simulink model "test_without_actuator"  (R2022b)
settings: Solver=FixedStepAuto  StartTime=0.0  StopTime=10  FixedStep=0.1  RelTol=1e-3
values from neighbouring files (symbols this model uses):
  C_M = 1.1366    [init.m]
  C_T = 3.5611    [init.m]
  D_p = 0.1    [init.m]
  model_param = struct(     'I', I,      'mass', ModelParam_m,      'g', ModelParam_g,      'c_T', ModelParam_c_T,      'c_M', ModelParam_c_M,      'd', ModelParam_d,      'J_RP', ModelParam_J_RP,      'init_pos', [ModelInit_Pos_x, ModelInit_Pos_y, ModelInit_Pos_z],      'init_att', [ModelInit_Att_x, ModelInit_Att_y, ModelInit_Att_z],      'C_T', C_T,      'C_M', C_M,      'air_density', p,      'prop_diameter',  ...(+52 chars)    [init.m]
  ModelInit_Att_qw = 0    [init.m]
  ModelInit_Att_qx = 1    [init.m]
  ModelInit_Att_qy = 0    [init.m]
  ModelInit_Att_qz = 0    [init.m]
  ModelInit_Pos_x = 0    [init.m]
  ModelInit_Pos_y = 0    [init.m]
  ModelInit_Pos_z = 0    [init.m]
  ModelParam_c_M = 1.779e-07*2    (= 3.558e-07)    [init.m]
  ModelParam_c_T = 1.105e-05    [init.m]
  ModelParam_d = 0.225    [init.m]
  ModelParam_g = 9.8    [init.m]
  ModelParam_I_xx = 0.0211    [init.m]
  ModelParam_I_yy = 0.0219    [init.m]
  ModelParam_I_zz = 0.0366    [init.m]
  ModelParam_J_RP = 0.0001287    [init.m]
  ModelParam_m = 1.4    [init.m]
  p = pos(idx,:)    [draw_morecool.m]    (also in init.m = 1.225)
(part 2 of 2)

== system test_without_actuator/混合无人机模型1/Quadcopter Dynamics Model/Rigid-Body Kinematic Model/Attitude Kinematic Model1 ==
  p : Inport
  q : Inport  Port=2
  r : Inport  Port=3
  Constant1 : Constant  Value=ModelInit_Att_qw
  Constant2 : Constant  Value=ModelInit_Att_qy
  Constant3 : Constant  Value=ModelInit_Att_qz
  Constant4 : Constant  Value=ModelInit_Att_qx
  Integrator{1,3..5} (4 alike) : Integrator  InitialConditionSource=external
  MATLAB Function1 : MATLAB Function  TreatAsAtomicUnit=on
  MATLAB Function2 : MATLAB Function  TreatAsAtomicUnit=on
  qw : Outport  VectorParamsAs1DForOutWhenUnconnected=off
  qx : Outport  Port=2  VectorParamsAs1DForOutWhenUnconnected=off
  qy : Outport  Port=3  VectorParamsAs1DForOutWhenUnconnected=off
  qz : Outport  Port=4  VectorParamsAs1DForOutWhenUnconnected=off
  wires:
  r/1 -> MATLAB Function2/3(r)
  MATLAB Function2/1(qw_dot) -> Integrator3/1
  q/1 -> MATLAB Function2/2(q)
  p/1 -> MATLAB Function2/1(p)
  Constant1/1 -> Integrator3/2
  Constant2/1 -> Integrator4/2
  Constant3/1 -> Integrator5/2
  MATLAB Function2/2(qx_dot) -> Integrator1/1
  Constant4/1 -> Integrator1/2
  MATLAB Function2/3(qy_dot) -> Integrator4/1
  MATLAB Function2/4(qz_dot) -> Integrator5/1
  Integrator3/1 -> MATLAB Function1/1(qw)
  Integrator1/1 -> MATLAB Function1/2(qx)
  Integrator4/1 -> MATLAB Function1/3(qy)
  Integrator5/1 -> MATLAB Function1/4(qz)
  MATLAB Function1/1(qw_unit) -> MATLAB Function2/4(qw), qw/1
  MATLAB Function1/2(qx_unit) -> MATLAB Function2/5(qx), qx/1
  MATLAB Function1/3(qy_unit) -> MATLAB Function2/6(qy), qy/1
  MATLAB Function1/4(qz_unit) -> MATLAB Function2/7(qz), qz/1

== system test_without_actuator/混合无人机模型1/Quadcopter Dynamics Model/Rigid-Body Kinematic Model/Position Kinematic Model ==
  v_x : Inport
  v_y : Inport  Port=2
  v_z : Inport  Port=3
  Constant1 : Constant  Value=ModelInit_Pos_z
  Constant2 : Constant  Value=ModelInit_Pos_y
  Constant3 : Constant  Value=ModelInit_Pos_x
  Integrator : Integrator  InitialConditionSource=external
  Integrator1 : Integrator  InitialConditionSource=external
  Integrator2 : Integrator  InitialConditionSource=external
  x : Outport  VectorParamsAs1DForOutWhenUnconnected=off
  y : Outport  Port=2  VectorParamsAs1DForOutWhenUnconnected=off
  z : Outport  Port=3  VectorParamsAs1DForOutWhenUnconnected=off
  wires:
  v_z/1 -> Integrator2/1
  Integrator1/1 -> y/1
  Integrator/1 -> x/1
  Constant1/1 -> Integrator2/2
  Integrator2/1 -> z/1
  v_x/1 -> Integrator/1
  v_y/1 -> Integrator1/1
  Constant2/1 -> Integrator1/2
  Constant3/1 -> Integrator/2

== system test_without_actuator/混合无人机模型2/Quadcopter Dynamics Model/Rigid-Body Dynamic Model/Attitude Dynamic Model ==
  tau_x : Inport
  tau_y : Inport  Port=2
  tau_z : Inport  Port=3
  w1 : Inport  Port=4
  w2 : Inport  Port=5
  w3 : Inport  Port=6
  w4 : Inport  Port=7
  Constant10 : Constant  Value=ModelParam_I_yy
  Constant11 : Constant  Value=ModelParam_I_zz
  Constant12 : Constant  Value=ModelParam_J_RP
  Constant9 : Constant  Value=ModelParam_I_xx
  Integrator10 : Integrator
  Integrator8 : Integrator
  Integrator9 : Integrator
  MATLAB Function : MATLAB Function  TreatAsAtomicUnit=on  SystemSampleTime=0.1
  Scope : Scope
  p : Outport  VectorParamsAs1DForOutWhenUnconnected=off
  q : Outport  Port=2  VectorParamsAs1DForOutWhenUnconnected=off
  r : Outport  Port=3  VectorParamsAs1DForOutWhenUnconnected=off
  wires:
  Constant9/1 -> MATLAB Function/8(I_xx)
  tau_z/1 -> MATLAB Function/3(tau_z)
  Integrator10/1 -> r/1, MATLAB Function/14(r)
  Constant12/1 -> MATLAB Function/11(J_RP)
  Integrator9/1 -> q/1, MATLAB Function/13(q)
  Constant10/1 -> MATLAB Function/9(I_yy)
  MATLAB Function/3(r_dot) -> Integrator10/1
  MATLAB Function/1(p_dot) -> Scope/1, Integrator8/1
  Integrator8/1 -> p/1, MATLAB Function/12(p)
  tau_y/1 -> MATLAB Function/2(tau_y)
  MATLAB Function/2(q_dot) -> Integrator9/1
  Constant11/1 -> MATLAB Function/10(I_zz)
  w1/1 -> MATLAB Function/4(w1)
  tau_x/1 -> MATLAB Function/1(tau_x)
  w2/1 -> MATLAB Function/5(w2)
  w3/1 -> MATLAB Function/6(w3)
  w4/1 -> MATLAB Function/7(w4)

== system test_without_actuator/混合无人机模型2/Quadcopter Dynamics Model/Rigid-Body Dynamic Model/Position Dynamic Model1 ==
  qw : Inport  SampleTime=0.1
  qx : Inport  Port=2
  qy : Inport  Port=3
  qz : Inport  Port=4
  f : Inport  Port=5
  Constant7 : Constant  Value=ModelParam_m  SampleTime=0.1
  Constant8 : Constant  Value=ModelParam_g  SampleTime=0.1
  Integrator1 : Integrator
  Integrator3 : Integrator
  Integrator6 : Integrator
  MATLAB Function : MATLAB Function  TreatAsAtomicUnit=on  SystemSampleTime=0.1
  v_x : Outport  VectorParamsAs1DForOutWhenUnconnected=off
  v_y : Outport  Port=2  VectorParamsAs1DForOutWhenUnconnected=off
  v_z : Outport  Port=3  VectorParamsAs1DForOutWhenUnconnected=off
  a_x : Outport  Port=4  VectorParamsAs1DForOutWhenUnconnected=off
  a_y : Outport  Port=5  VectorParamsAs1DForOutWhenUnconnected=off
  a_z : Outport  Port=6  VectorParamsAs1DForOutWhenUnconnected=off
  wires:
  Constant8/1 -> MATLAB Function/2(g)
  MATLAB Function/1(v_x_dot) -> a_x/1, Integrator6/1
  MATLAB Function/2(v_y_dot) -> a_y/1, Integrator1/1
  qx/1 -> MATLAB Function/4(qx)
  Constant7/1 -> MATLAB Function/1(m)
  MATLAB Function/3(v_z_dot) -> a_z/1, Integrator3/1
  qw/1 -> MATLAB Function/3(qw)
  f/1 -> MATLAB Function/7(f)
  qy/1 -> MATLAB Function/5(qy)
  Integrator6/1 -> v_x/1
  Integrator1/1 -> v_y/1
  Integrator3/1 -> v_z/1
  qz/1 -> MATLAB Function/6(qz)

== system test_without_actuator/混合无人机模型2/Quadcopter Dynamics Model/Rigid-Body Kinematic Model/Attitude Kinematic Model1 ==
  p : Inport
  q : Inport  Port=2
  r : Inport  Port=3
  Constant1 : Constant  Value=ModelInit_Att_qw
  Constant2 : Constant  Value=ModelInit_Att_qy
  Constant3 : Constant  Value=ModelInit_Att_qz
  Constant4 : Constant  Value=ModelInit_Att_qx
  Integrator{1,3..5} (4 alike) : Integrator  InitialConditionSource=external
  MATLAB Function1 : MATLAB Function  TreatAsAtomicUnit=on
  MATLAB Function2 : MATLAB Function  TreatAsAtomicUnit=on
  qw : Outport  VectorParamsAs1DForOutWhenUnconnected=off
  qx : Outport  Port=2  VectorParamsAs1DForOutWhenUnconnected=off
  qy : Outport  Port=3  VectorParamsAs1DForOutWhenUnconnected=off
  qz : Outport  Port=4  VectorParamsAs1DForOutWhenUnconnected=off
  wires:
  r/1 -> MATLAB Function2/3(r)
  MATLAB Function2/1(qw_dot) -> Integrator3/1
  q/1 -> MATLAB Function2/2(q)
  p/1 -> MATLAB Function2/1(p)
  Constant1/1 -> Integrator3/2
  Constant2/1 -> Integrator4/2
  Constant3/1 -> Integrator5/2
  MATLAB Function2/2(qx_dot) -> Integrator1/1
  Constant4/1 -> Integrator1/2
  MATLAB Function2/3(qy_dot) -> Integrator4/1
  MATLAB Function2/4(qz_dot) -> Integrator5/1
  Integrator3/1 -> MATLAB Function1/1(qw)
  Integrator1/1 -> MATLAB Function1/2(qx)
  Integrator4/1 -> MATLAB Function1/3(qy)
  Integrator5/1 -> MATLAB Function1/4(qz)
  MATLAB Function1/1(qw_unit) -> MATLAB Function2/4(qw), qw/1
  MATLAB Function1/2(qx_unit) -> MATLAB Function2/5(qx), qx/1
  MATLAB Function1/3(qy_unit) -> MATLAB Function2/6(qy), qy/1
  MATLAB Function1/4(qz_unit) -> MATLAB Function2/7(qz), qz/1

== system test_without_actuator/混合无人机模型2/Quadcopter Dynamics Model/Rigid-Body Kinematic Model/Position Kinematic Model ==
  v_x : Inport
  v_y : Inport  Port=2
  v_z : Inport  Port=3
  Constant1 : Constant  Value=ModelInit_Pos_z
  Constant2 : Constant  Value=ModelInit_Pos_y
  Constant3 : Constant  Value=ModelInit_Pos_x
  Integrator : Integrator  InitialConditionSource=external
  Integrator1 : Integrator  InitialConditionSource=external
  Integrator2 : Integrator  InitialConditionSource=external
  x : Outport  VectorParamsAs1DForOutWhenUnconnected=off
  y : Outport  Port=2  VectorParamsAs1DForOutWhenUnconnected=off
  z : Outport  Port=3  VectorParamsAs1DForOutWhenUnconnected=off
  wires:
  v_z/1 -> Integrator2/1
  Integrator1/1 -> y/1
  Integrator/1 -> x/1
  Constant1/1 -> Integrator2/2
  Integrator2/1 -> z/1
  v_x/1 -> Integrator/1
  v_y/1 -> Integrator1/1
  Constant2/1 -> Integrator1/2
  Constant3/1 -> Integrator/2

== matlab function test_without_actuator/混合无人机模型1/Quadcopter Dynamics Model/Rigid-Body Dynamic Model/Position Dynamic Model1/MATLAB Function ==
  data: m input; g input; qw input; qx input; qy input; qz input; f input; v_x_dot output; v_y_dot output; v_z_dot output
function [v_x_dot, v_y_dot, v_z_dot] = fcn(m, g, qw, qx, qy, qz, f)
% 函数描述
% 1.作用：本函数为四旋翼的位置动力学微分方程组，通过四旋翼所受拉力、姿态角
%         计算得到四旋翼飞行器的加速度
% 2.函数输入：
%   m：四旋翼飞行器质量(kg)
%   g：重力加速度(m/s^2)
%   qw：四元数1号位
%   qx：四元数2号位
%   qy：四元数3号位
%   qz：四元数4号位
%   f：螺旋桨产生的总拉力(N)
% 3.函数输出：
%   v_x_dot：地球坐标系下沿x轴的速度的导数
%   v_y_dot：地球坐标系下沿y轴的速度的导数
%   v_z_dot：地球坐标系下沿z轴的速度的导数
% 4.四旋翼构型为"+”型，螺旋桨序号如下所示：
%            y
%            2↑
%            |
%        3↓—— —— 1↓   x
%            |
%            4↑
%   其中，↑表示螺旋桨逆时针旋转；↓表示螺旋桨顺时针旋转。
% 计算旋转矩阵 R
R11 = 1 - 2*qy^2 - 2*qz^2;
R12 = 2*qx*qy - 2*qz*qw;
R13 = 2*qx*qz + 2*qy*qw;
R21 = 2*qx*qy + 2*qz*qw;
R22 = 1 - 2*qx^2 - 2*qz^2;
R23 = 2*qy*qz - 2*qx*qw;
R31 = 2*qx*qz - 2*qy*qw;
R32 = 2*qy*qz + 2*qx*qw;
R33 = 1 - 2*qx^2 - 2*qy^2;

v_x_dot = f * (1/m) * (R13);
v_y_dot = f * (1/m) * (R23);
v_z_dot = f * (1/m) * R33 - g;
end

== matlab function test_without_actuator/混合无人机模型1/Quadcopter Dynamics Model/Rigid-Body Kinematic Model/Attitude Kinematic Model1/MATLAB Function1 ==
  data: qw_unit output; qw input; qx input; qy input; qz input; qx_unit output; qy_unit output; qz_unit output
function [qw_unit, qx_unit, qy_unit, qz_unit] = normalize_quaternion(qw, qx, qy, qz)
    % 计算四元数的模
    norm_q = sqrt(qw^2 + qx^2 + qy^2 + qz^2);
    
    % 检查模是否为零，避免除以零的错误
    if norm_q == 0
        error('Zero norm quaternion cannot be normalized.');
    end

    % 单位化四元数
    qw_unit = qw / norm_q;
    qx_unit = qx / norm_q;
    qy_unit = qy / norm_q;
    qz_unit = qz / norm_q;
end

== matlab function test_without_actuator/混合无人机模型1/Quadcopter Dynamics Model/Rigid-Body Kinematic Model/Attitude Kinematic Model1/MATLAB Function2 ==
  data: p input; qw_dot output; q input; r input; qw input; qx input; qy input; qz input; qx_dot output; qy_dot output; qz_dot output
function [qw_dot, qx_dot, qy_dot, qz_dot] = updateQuaternion(p, q, r, qw, qx, qy, qz)
    % updateQuaternion 更新无人机的姿态四元数
    % 输入:
    %   q - 当前姿态四元数，形式为 [qw, qx, qy, qz]
    %   omega - 三轴角速度，形式为 [omega_x, omega_y, omega_z]
    %   dt - 时间步长

    % 将角速度转换为四元数形式
    q_current = [qw, qx, qy, qz];
    omega_q = [0, p, q, r];
    
    % 计算四元数的导数
    q_dot = 0.5 * quatmultiply(omega_q, q_current);
    qw_dot = q_dot(1);
    qx_dot = q_dot(2);
    qy_dot = q_dot(3);
    qz_dot = q_dot(4);
end

== matlab function test_without_actuator/混合无人机模型2/Quadcopter Dynamics Model/MATLAB Function ==
  data: x input; density output; y input
function density = air_density(x, y)
    % 定义火坑的中心位置
    center_x = 10;
    center_y = 10;

    % 定义火坑的半径
    radius = 0.00001;

    % 定义火坑中心的空气密度为1.078 kg/m³
    density_center = 1.078;

    % 定义火坑边缘的空气密度为日常密度值
    density_edge = 1.225;

    % 计算无人机到火坑中心的距离
    r = sqrt((x - center_x)^2 + (y - center_y)^2);

    % 定义高斯函数的标准差
    sigma = radius / 3;
    
    % 使用高斯函数计算空气密度
    density = density_edge + (density_center - density_edge) * exp(-(r.^2) / (2 * sigma^2));


    density = density/1.225;
end

== matlab function test_without_actuator/混合无人机模型2/Quadcopter Dynamics Model/Rigid-Body Dynamic Model/Attitude Dynamic Model/MATLAB Function ==
  data: tau_x input; p_dot output; tau_y input; tau_z input; w1 input; w2 input; w3 input; w4 input; I_xx input; I_yy input; I_zz input; J_RP input; p input; q input; r input; q_dot output; r_dot output
function [p_dot, q_dot, r_dot] = fcn(tau_x, tau_y, tau_z, w1, w2, w3, w4, I_xx, I_yy, I_zz, J_RP, p, q, r)
% 函数描述
% 1.作用：本函数为四旋翼的姿态动力学微分方程组，通过四旋翼所受力矩和螺旋
%         桨转速计算得到四旋翼的机体角速度
% 2.函数输入：
%   wi：四个螺旋桨的转速(rad/s)
%   tau_x：x轴反扭力矩（机体轴）(N·m)
%   tau_y：y轴反扭力矩（机体轴）(N·m)
%   tau_z：z轴反扭力矩（机体轴）(N·m)
%   I_xx：四旋翼x轴转动惯量(kg·m^2)
%   I_yy：四旋翼y轴转动惯量(kg·m^2)
%   I_zz：四旋翼z轴转动惯量(kg·m^2)
%   J_RP：整个电机转子和螺旋桨绕转轴的总转动惯量(kg·m^2)
%   p：四旋翼x轴角速度（机体轴)(rad/s)
%   q：四旋翼y轴角速度（机体轴)(rad/s)
%   r：四旋翼z轴角速度（机体轴)(rad/s)
% 3.函数输出：
%   p_dot：四旋翼x轴角加速度（机体轴)
%   q_dot：四旋翼y轴角加速度（机体轴)
%   r_dot：四旋翼z轴角加速度（机体轴)
% 4.四旋翼构型为“X”型，螺旋桨序号如下所示：
%            y
%            2↑
%            |
%        3↓—— —— 1↓   x
%            |
%            4↑
%   其中，↑表示螺旋桨逆时针旋转；↓表示螺旋桨顺时针旋转。


p_dot = (1/I_xx) * (tau_x + q * r * (I_yy - I_zz) );
q_dot = (1/I_yy) * (tau_y + p * r * (I_zz - I_xx) );
r_dot = (1/I_zz) * (tau_z + p * q * (I_xx - I_yy) );
end

== matlab function test_without_actuator/混合无人机模型2/Quadcopter Dynamics Model/Rigid-Body Dynamic Model/Position Dynamic Model1/MATLAB Function ==
  data: m input; g input; qw input; qx input; qy input; qz input; f input; v_x_dot output; v_y_dot output; v_z_dot output
function [v_x_dot, v_y_dot, v_z_dot] = fcn(m, g, qw, qx, qy, qz, f)
% 函数描述
% 1.作用：本函数为四旋翼的位置动力学微分方程组，通过四旋翼所受拉力、姿态角
%         计算得到四旋翼飞行器的加速度
% 2.函数输入：
%   m：四旋翼飞行器质量(kg)
%   g：重力加速度(m/s^2)
%   qw：四元数1号位
%   qx：四元数2号位
%   qy：四元数3号位
%   qz：四元数4号位
%   f：螺旋桨产生的总拉力(N)
% 3.函数输出：
%   v_x_dot：地球坐标系下沿x轴的速度的导数
%   v_y_dot：地球坐标系下沿y轴的速度的导数
%   v_z_dot：地球坐标系下沿z轴的速度的导数
% 4.四旋翼构型为"+”型，螺旋桨序号如下所示：
%            y
%            2↑
%            |
%        3↓—— —— 1↓   x
%            |
%            4↑
%   其中，↑表示螺旋桨逆时针旋转；↓表示螺旋桨顺时针旋转。
% 计算旋转矩阵 R
R11 = 1 - 2*qy^2 - 2*qz^2;
R12 = 2*qx*qy - 2*qz*qw;
R13 = 2*qx*qz + 2*qy*qw
R21 = 2*qx*qy + 2*qz*qw;
R22 = 1 - 2*qx^2 - 2*qz^2;
R23 = 2*qy*qz - 2*qx*qw
R31 = 2*qx*qz - 2*qy*qw;
R32 = 2*qy*qz + 2*qx*qw;
R33 = 1 - 2*qx^2 - 2*qy^2

v_x_dot = f * (1/m) * (R13)
v_y_dot = f * (1/m) * (R23)
v_z_dot = f * (1/m) * R33 - g
end

== matlab function test_without_actuator/混合无人机模型2/Quadcopter Dynamics Model/Rigid-Body Kinematic Model/Attitude Kinematic Model1/MATLAB Function1 ==
  data: qw_unit output; qw input; qx input; qy input; qz input; qx_unit output; qy_unit output; qz_unit output
function [qw_unit, qx_unit, qy_unit, qz_unit] = normalize_quaternion(qw, qx, qy, qz)
    % 计算四元数的模
    norm_q = sqrt(qw^2 + qx^2 + qy^2 + qz^2);
    
    % 检查模是否为零，避免除以零的错误
    if norm_q == 0
        error('Zero norm quaternion cannot be normalized.');
    end

    % 单位化四元数
    qw_unit = qw / norm_q;
    qx_unit = qx / norm_q;
    qy_unit = qy / norm_q;
    qz_unit = qz / norm_q;
end

== matlab function test_without_actuator/混合无人机模型2/Quadcopter Dynamics Model/Rigid-Body Kinematic Model/Attitude Kinematic Model1/MATLAB Function2 ==
  data: p input; qw_dot output; q input; r input; qw input; qx input; qy input; qz input; qx_dot output; qy_dot output; qz_dot output
function [qw_dot, qx_dot, qy_dot, qz_dot] = updateQuaternion(p, q, r, qw, qx, qy, qz)
    % updateQuaternion 更新无人机的姿态四元数
    % 输入:
    %   q - 当前姿态四元数，形式为 [qw, qx, qy, qz]
    %   omega - 三轴角速度，形式为 [omega_x, omega_y, omega_z]
    %   dt - 时间步长

    % 将角速度转换为四元数形式
    q_current = [qw, qx, qy, qz];
    omega_q = [0, p, q, r];
    
    % 计算四元数的导数
    q_dot = 0.5 * quatmultiply(omega_q, q_current);
    qw_dot = q_dot(1);
    qx_dot = q_dot(2);
    qy_dot = q_dot(3);
    qz_dot = q_dot(4);
end

== matlab function test_without_actuator/MATLAB Function1 ==
  data: f input; w1 output; tau_x input; tau_y input; w2 output; w3 output; tau_z input; w4 output; C_T input; C_M input; p input; D_p input; D input
function [w1, w2, w3, w4] = converter(f, tau_x, tau_y, tau_z, C_T, C_M, p, D_p, D)
    % 初始化旋翼转速
    w1 = 0;
    w2 = 0;
    w3 = 0;
    w4 = 0;

    % 转换力和力矩到旋翼转速
    % 所需参数：推力系数 C_T，力矩系数 C_M，空气密度 ρ，螺旋桨直径 D_p，UAV 臂长 D
    % 输入力和力矩
    a = [f; tau_x; tau_y; tau_z];

    % 计算推力和力矩转换矩阵
    KF = C_T * p * D_p^4 / (4 * pi^2);
    KM = C_M * p * D_p^5 / (4 * pi^2);
    A = [KF, KF, KF, KF;
         0, KF * D, 0, -KF * D;
         -KF * D, 0, KF * D, 0;
         KM, -KM, KM, -KM];

    % 求解方程 Ax = b
    b = A \ a; % 求解向量 b
    
    % 直接分配旋翼速度，允许负值
    w1 = sign(b(1)) * sqrt(abs(b(1)));
    w2 = sign(b(2)) * sqrt(abs(b(2)));
    w3 = sign(b(3)) * sqrt(abs(b(3)));
    w4 = sign(b(4)) * sqrt(abs(b(4)));
end

== matlab function test_without_actuator/混合无人机模型/Quadcopter Dynamics Model/Control Effectiveness Model/MATLAB Function ==
  data: w1 input; f output; w2 input; w3 input; w4 input; c_T input; c_M input; d input; tau_x output; tau_y output; tau_z output; p input; Eta input
function [f, tau_x, tau_y, tau_z] = fcn(w1, w2, w3, w4, c_T, c_M, d, p, Eta)
% 函数描述
% 1.作用：本函数用来计算螺旋桨旋转产生的总拉力和反扭力矩。
% 2.函数输入：
%   wi：四个螺旋桨的转速(rad/s)，可以为正或负
%   c_T：螺旋桨拉力系数和外面的converter的CT不同，已经经过换算就等于KF
%   c_M：螺旋桨转矩系数= KM
%   d：机体中心和任一电机的距离(m)
% 3.函数输出：
%   f：螺旋桨拉力（机体轴）
%   tau_x：x轴反扭力矩（机体轴）
%   tau_y：y轴反扭力矩（机体轴）
%   tau_z：z轴反扭力矩（机体轴）
% 4.四旋翼构型为“X”型

% 计算每个螺旋桨产生的推力影响，考虑转速正负
f = p*c_T * (sign(w1)*w1^2 + sign(w2)*w2^2 + sign(w3)*w3^2 + sign(w4)*w4^2);
% 计算x轴扭矩，考虑螺旋桨的位置和旋转方向
tau_x = p*d * c_T * (-w2^2 + w4^2);
% 计算y轴扭矩
tau_y = p*d * c_T * (-w1^2 + w3^2);
% 计算z轴扭矩，只考虑螺旋桨转速和旋转方向
tau_z = p*c_M * (sign(w1)*w1^2 - sign(w2)*w2^2 + sign(w3)*w3^2 - sign(w4)*w4^2);

% 计算每个螺旋桨产生的推力影响，考虑转速正负
f = p*c_T * (w1^2 + w2^2 + w3^2 + w4^2);
% 计算x轴扭矩，考虑螺旋桨的位置和旋转方向
tau_x = p*d * c_T * (-w2^2 + w4^2);
% 计算y轴扭矩
tau_y = p*d * c_T * (-w1^2 + w3^2);
% 计算z轴扭矩，只考虑螺旋桨转速和旋转方向
tau_z = p*c_M * (w1^2 - w2^2 + w3^2 - w4^2);
f = -f;
  

end

== matlab function test_without_actuator/混合无人机模型/Quadcopter Dynamics Model/MATLAB Function ==
  data: x input; density output; y input
function density = air_density(x, y)
    % 定义火坑的中心位置
    center_x = 10;
    center_y = 10;

    % 定义火坑的半径
    radius = 0.00001;

    % 定义火坑中心的空气密度为1.078 kg/m³
    density_center = 1.078;

    % 定义火坑边缘的空气密度为日常密度值
    density_edge = 1.225;

    % 计算无人机到火坑中心的距离
    r = sqrt((x - center_x)^2 + (y - center_y)^2);

    % 定义高斯函数的标准差
    sigma = radius / 3;
    
    % 使用高斯函数计算空气密度
    density = density_edge + (density_center - density_edge) * exp(-(r.^2) / (2 * sigma^2));


    density = density/1.225;
end

== matlab function test_without_actuator/混合无人机模型/Quadcopter Dynamics Model/Rigid-Body Dynamic Model/Attitude Dynamic Model/MATLAB Function ==
  data: tau_x input; p_dot output; tau_y input; tau_z input; w1 input; w2 input; w3 input; w4 input; I_xx input; I_yy input; I_zz input; J_RP input; p input; q input; r input; q_dot output; r_dot output
function [p_dot, q_dot, r_dot] = fcn(tau_x, tau_y, tau_z, w1, w2, w3, w4, I_xx, I_yy, I_zz, J_RP, p, q, r)
% 函数描述
% 1.作用：本函数为四旋翼的姿态动力学微分方程组，通过四旋翼所受力矩和螺旋
%         桨转速计算得到四旋翼的机体角速度
% 2.函数输入：
%   wi：四个螺旋桨的转速(rad/s)
%   tau_x：x轴反扭力矩（机体轴）(N·m)
%   tau_y：y轴反扭力矩（机体轴）(N·m)
%   tau_z：z轴反扭力矩（机体轴）(N·m)
%   I_xx：四旋翼x轴转动惯量(kg·m^2)
%   I_yy：四旋翼y轴转动惯量(kg·m^2)
%   I_zz：四旋翼z轴转动惯量(kg·m^2)
%   J_RP：整个电机转子和螺旋桨绕转轴的总转动惯量(kg·m^2)
%   p：四旋翼x轴角速度（机体轴)(rad/s)
%   q：四旋翼y轴角速度（机体轴)(rad/s)
%   r：四旋翼z轴角速度（机体轴)(rad/s)
% 3.函数输出：
%   p_dot：四旋翼x轴角加速度（机体轴)
%   q_dot：四旋翼y轴角加速度（机体轴)
%   r_dot：四旋翼z轴角加速度（机体轴)
% 4.四旋翼构型为“X”型，螺旋桨序号如下所示：
%            y
%            2↑
%            |
%        3↓—— —— 1↓   x
%            |
%            4↑
%   其中，↑表示螺旋桨逆时针旋转；↓表示螺旋桨顺时针旋转。

Omega = w1 - w2 + w3 - w4;
p_dot = (1/I_xx) * (tau_x + q * r * (I_yy - I_zz) - J_RP * q * Omega);
q_dot = (1/I_yy) * (tau_y + p * r * (I_zz - I_xx) + J_RP * p * Omega);
r_dot = (1/I_zz) * (tau_z + p * q * (I_xx - I_yy) );
end

== matlab function test_without_actuator/混合无人机模型/Quadcopter Dynamics Model/Rigid-Body Dynamic Model/Position Dynamic Model1/MATLAB Function ==
  data: m input; g input; qw input; qx input; qy input; qz input; f input; v_x_dot output; v_y_dot output; v_z_dot output
function [v_x_dot, v_y_dot, v_z_dot] = fcn(m, g, qw, qx, qy, qz, f)
% 函数描述
% 1.作用：本函数为四旋翼的位置动力学微分方程组，通过四旋翼所受拉力、姿态角
%         计算得到四旋翼飞行器的加速度
% 2.函数输入：
%   m：四旋翼飞行器质量(kg)
%   g：重力加速度(m/s^2)
%   qw：四元数1号位
%   qx：四元数2号位
%   qy：四元数3号位
%   qz：四元数4号位
%   f：螺旋桨产生的总拉力(N)
% 3.函数输出：
%   v_x_dot：地球坐标系下沿x轴的速度的导数
%   v_y_dot：地球坐标系下沿y轴的速度的导数
%   v_z_dot：地球坐标系下沿z轴的速度的导数
% 4.四旋翼构型为"+”型，螺旋桨序号如下所示：
%            y
%            2↑
%            |
%        3↓—— —— 1↓   x
%            |
%            4↑
%   其中，↑表示螺旋桨逆时针旋转；↓表示螺旋桨顺时针旋转。
% 计算旋转矩阵 R
R11 = 1 - 2*qy^2 - 2*qz^2;
R12 = 2*qx*qy - 2*qz*qw;
R13 = 2*qx*qz + 2*qy*qw;
R21 = 2*qx*qy + 2*qz*qw;
R22 = 1 - 2*qx^2 - 2*qz^2;
R23 = 2*qy*qz - 2*qx*qw;
R31 = 2*qx*qz - 2*qy*qw;
R32 = 2*qy*qz + 2*qx*qw;
R33 = 1 - 2*qx^2 - 2*qy^2;

v_x_dot = f * (1/m) * (R13);
v_y_dot = f * (1/m) * (R23);
v_z_dot = f * (1/m) * R33 - g;
end

== matlab function test_without_actuator/混合无人机模型/Quadcopter Dynamics Model/Rigid-Body Kinematic Model/Attitude Kinematic Model1/MATLAB Function1 ==
  data: qw_unit output; qw input; qx input; qy input; qz input; qx_unit output; qy_unit output; qz_unit output
function [qw_unit, qx_unit, qy_unit, qz_unit] = normalize_quaternion(qw, qx, qy, qz)
    % 计算四元数的模
    norm_q = sqrt(qw^2 + qx^2 + qy^2 + qz^2);
    
    % 检查模是否为零，避免除以零的错误
    if norm_q == 0
        error('Zero norm quaternion cannot be normalized.');
    end

    % 单位化四元数
    qw_unit = qw / norm_q;
    qx_unit = qx / norm_q;
    qy_unit = qy / norm_q;
    qz_unit = qz / norm_q;
end

== matlab function test_without_actuator/混合无人机模型/Quadcopter Dynamics Model/Rigid-Body Kinematic Model/Attitude Kinematic Model1/MATLAB Function2 ==
  data: p input; qw_dot output; q input; r input; qw input; qx input; qy input; qz input; qx_dot output; qy_dot output; qz_dot output
function [qw_dot, qx_dot, qy_dot, qz_dot] = updateQuaternion(p, q, r, qw, qx, qy, qz)
    % updateQuaternion 更新无人机的姿态四元数
    % 输入:
    %   q - 当前姿态四元数，形式为 [qw, qx, qy, qz]
    %   omega - 三轴角速度，形式为 [omega_x, omega_y, omega_z]
    %   dt - 时间步长

    % 将角速度转换为四元数形式
    q_current = [qw, qx, qy, qz];
    omega_q = [0, p, q, r];
    
    % 计算四元数的导数
    q_dot = 0.5 * quatmultiply(omega_q, q_current);
    qw_dot = q_dot(1);
    qx_dot = q_dot(2);
    qy_dot = q_dot(3);
    qz_dot = q_dot(4);
end

== matlab function test_without_actuator/MATLAB Function5 ==
  data: current_state input; u1 output; desired_state input; model_param input; u2 output; u3 output; K input; u4 output; Eta input
function [u1, u2, u3, u4] = controller(current_state, desired_state, model_param, K, Eta)
%disp('fuck2')

J = model_param.I; % Moment of inertia wrt body frame

% position error
ep = current_state(1:3)-desired_state.pos;

% velocity error
ev = current_state(4:6)-desired_state.vel;

% desired force, F_des
Kp = K.Kp;
Kv = K.Kv;
KR = K.KR;
K_omega = K.K_omega;
m = model_param.mass;
g = model_param.g;
acc  = -Kp*ep -Kv*ev + g*[0 0 1]' + desired_state.acc;
Fd = m*acc
%Fd = -Kp*ep -Kv*ev + m*g*[0 0 1]' + m*desired_state.acc;

% desired input u1
qw = current_state(7);
qx = current_state(8);
qy = current_state(9);
qz = current_state(10);
R = qToR(qw, qx, qy, qz) % Current rotation，（当前姿态也许需要换成四元数形式√）
% current z-axis in body frame
zb = R(:,3);%R的每一列都是单位向量

u1 = Fd'*zb;%计算无人机提供的期望推力
%Fd、zb是世界坐标系
current_acc = -g*[0 0 1]'+u1*zb;
%if的条件不应是NS而应该是+-
%实际上控制量u1的正负就可以代替Eta指示推力正负，此时不需要提前指示Eta的正负，但是还需要加入推力变化的过渡过程。
%即Eta在位置控制中无影响？
%新问题是如果控制器自行选择
if zb(3)>=0 && Eta == 1
%if Eta == 1
    u1 = Fd'*zb
    current_acc = -g*[0 0 1]'+u1*zb;
end
if zb(3)>=0 && Eta == -1
%if Eta == 1
    %u1 = Fd'*(-zb)
    u1 = Fd'*(zb)
    current_acc = -g*[0 0 1]'+u1*(-zb);
end
if zb(3)<0 && Eta == 1
%if Eta == 1
    u1 = Fd'*zb
    current_acc = -g*[0 0 1]'+u1*zb;
end
if zb(3)<0 && Eta == -1
%if Eta == -1
    %u1 = Fd'*(-zb)
    u1 = Fd'*(zb)
    current_acc = -g*[0 0 1]'+u1*(-zb);
end
%——————————————————————————————————————上面是位置控制器——————————————————————————————————————
%——————————————————————————————————————下面是姿态控制器——————————————————————————————————————


% accel error
ea = current_acc-desired_state.acc;
% Desired force derivative
acc_dot = -Kp*ev -Kv*ea + desired_state.jerk;
Fd_dot = m*acc_dot;
%?????????????！！！！！！！！！！！！！！！！！！！！！！！！！！！！！！！！！！！！！！！！！
% desired rotation, Rd = [xbd ybd zbd]
zbd = acc/norm(acc);
a = zbd(1);
b = zbd(2);
c = zbd(3);
if Eta == 1
    zbd = acc/norm(acc)
    a = zbd(1);
    b = zbd(2);
    c = zbd(3);
end
if Eta == -1
    zbd = -acc/norm(acc)
    a = zbd(1);
    b = zbd(2);
    c = zbd(3);
end
Mode = switchMode([a,b,c]);
%还要算abc的导数 检查这里！！！！！！！！！！！！！！！！！！！！！！！！！！！！！！！！！！！可能因为上面的分类讨论导致abc的导数表示形式不同
a_dot=0;b_dot=0;c_dot=0;I=eye(3);
if Eta == 1
    %Fd_norm_dot = Fd'*Fd_dot/norm(Fd);
    %zbd_dot = (Fd_dot*norm(Fd) - Fd*Fd_norm_dot)/norm(Fd)^2;
    zbd_dot = (acc'*acc*I-acc*acc')*acc_dot/(norm(acc))^3;
    a_dot = zbd_dot(1);
    b_dot = zbd_dot(2);
    c_dot = zbd_dot(3);
end
if Eta == -1
    zbd_dot = -(acc'*acc*I-acc*acc')*acc_dot/(norm(acc))^3;
    a_dot = zbd_dot(1);
    b_dot = zbd_dot(2);
    c_dot = zbd_dot(3);
end
% ybd = zbd X xcd/norm(zbd X xcd)
% xcd
% 模式N
yawd = desired_state.yaw;
yawd_dot = desired_state.yawdot;
yawd_2dot = desired_state.yawddot;
% 模式S
yawd_1 = 2*atan2(a,b) + yawd;
%if yawd_1>= 2*pi
%    yawd_1 = yawd_1 - 2*pi;
%end
%yawd_1_dot = (a_dot*b-a*b_dot)/(a^2+b^2)
if a == 0&&b == 0
    yawd_1_dot = 0;  %或者定义一个其他合理的值
else
    yawd_1_dot = 2*(a_dot * b - a * b_dot) / (a^2 + b^2);
end
%-------------------------------------------------------------------------------------必要素材已经准备好，r、ψ->a、b、c、ψ
%期望姿态Rd、姿态误差eR
u2 = 0; u3 = 0; u4 = 0; % 默认值
if Mode == 'N'
    q_1 = q_abc(a,b,c);
    q_2 = q_psi(yawd);
    q_3 = quatmultiply(q_1, q_2)
    Rd = qToR(q_3(1), q_3(2), q_3(3), q_3(4))
    R1 = (Rd'*R - R'*Rd)
    q = [qw,qx,qy,qz];
    %eR = 1/2*vee_optr(R1)
    eR = calculateAttitudeError(q,q_3)
    %期望角速度wd、角速度误差ew
    current_omega = current_state(11:13);
    wd = [sin(yawd)*a_dot - cos(yawd)*b_dot - (a*sin(yawd)-b*cos(yawd))*(c_dot/(c+1));
          cos(yawd)*a_dot + sin(yawd)*b_dot - (a*cos(yawd)+b*sin(yawd))*(c_dot/(c+1));
          (b*a_dot-a*b_dot)/(1+c)+yawd_dot];
    ew = current_omega - R'*Rd*wd;
    M = -KR*eR -K_omega*ew;
    u2 = M(1);u3 = M(2); u4 = M(3);
end

if Mode == 'S'
    q_1 = q_abc_1(a,b,c);
    q_2 = q_psi(yawd);
    q_3 = quatmultiply(q_1, q_2);
    Rd = qToR(q_3(1), q_3(2), q_3(3), q_3(4))
    R1 = (Rd'*R - R'*Rd);
    q = [qw,qx,qy,qz];
    %eR = 1/2*vee_optr(R1)
    eR = calculateAttitudeError(q,q_3)
    %期望角速度wd、角速度误差ew
    current_omega = current_state(11:13);
    wd = [sin(yawd_1)*a_dot + cos(yawd_1)*b_dot - (a*sin(yawd_1)+b*cos(yawd_1))*(c_dot/(c-1));
          cos(yawd_1)*a_dot - sin(yawd_1)*b_dot - (a*cos(yawd_1)-b*sin(yawd_1))*(c_dot/(c-1));
          (b*a_dot-a*b_dot)/(-1+c)+yawd_1_dot];
    ew = current_omega - R'*Rd*wd;
    M = -KR*eR -K_omega*ew;
    u2 = M(1);
    u3 = M(2);
    u4 = M(3);
end
%--------------------------------------------------------------------------------------------------------over！
% xcd = [cos(yawd) sin(yawd) 0]';
% ybd = hat_optr(zbd)*xcd/norm(hat_optr(zbd)*xcd);%hat_optr用于向量叉乘
% % xbd = ybd X zbd
% xbd = hat_optr(ybd)*zbd;
% Rd1 = [xbd ybd zbd];
% %————————————————————————————————原版计算期望姿态R的方式过于复杂，现在直接有了期望四元数的参数化(a,b,c)
% % 而(a,b,c)又可以被表示为加速度a(来自于推力和z轴平行），进而表示为r的二阶导数
% Rd2 = [-xbd -ybd zbd];
% 
% % eR orientation error
% R1 = (Rd1'*R - R'*Rd1);
% R2 = (Rd2'*R - R'*Rd2);
% 
% eR1 = 1/2*vee_optr(R1);%vee_optr用于将反对称矩阵变回向量，是hat的逆操作
% eR2 = 1/2*vee_optr(R2);
% % if norm(eR1) >= norm(eR2)
% %     Rd = Rd2;
% %     eR = eR2;
% %     xbd = -xbd;
% %     ybd = -ybd;
% % else
%     Rd = Rd1;
%     eR = eR1;
% % end
% 
% current_omega = current_state(23:25);
% 
% % Desired omega^ = Rd'*R
% Fd_norm_dot = Fd'*Fd_dot/norm(Fd);
% zbd_dot = (Fd_dot*norm(Fd) - Fd*Fd_norm_dot)/norm(Fd)^2;
% xcd_dot = [-sin(yawd) cos(yawd) 0]'*desired_state.yawdot;
% 
% zbd_x_xcd_dot = hat_optr(zbd_dot)*xcd + hat_optr(zbd)*xcd_dot;
% zbd_xcd_norm_dot = (hat_optr(zbd)*xcd)'*(zbd_x_xcd_dot)/norm(hat_optr(zbd)*xcd);
% 
% 
% ybd_dot = (zbd_x_xcd_dot*norm(hat_optr(zbd)*xcd) - hat_optr(zbd)*xcd*zbd_xcd_norm_dot)/norm(hat_optr(zbd)*xcd)^2;
% xbd_dot = hat_optr(ybd_dot)*zbd + hat_optr(ybd)*zbd_dot;
% 
% Rd_dot = [xbd_dot ybd_dot zbd_dot];
% wd_hat = Rd'*Rd_dot;
% wd = vee_optr(wd_hat);
% % error
% ew = current_omega - R'*Rd*wd;
% 
% % Desired angular accerelation^ = Rd_dot'*Rd_dot + Rd'*Rd_2dot;
% R_dot = R*hat_optr(current_omega);
% zb_dot = R_dot(:,3);
% u1_dot = Fd_dot'*zb + Fd'*zb_dot;
% current_jerk = (u1_dot*zb + u1*zb_dot)/m;
% ej = current_jerk - desired_state.jerk;
% Fd_2dot = -Kp*ea -Kv*ej + m*desired_state.snap;
% zbd_2dot = (Fd_2dot*norm(Fd)-Fd_dot*Fd_norm_dot)/norm(Fd)^2 -...
%            (((Fd_dot'*Fd_dot + Fd'*Fd_2dot)*Fd + (Fd'*Fd_dot)*Fd_dot)*norm(Fd)^3 -...
%            (Fd'*Fd_dot)*Fd * 3*norm(Fd)*(Fd'*Fd_dot))/norm(Fd)^4;
% 
% % ybd_2dot
% xcd_2dot = [-cos(yawd)*yawd_dot^2-sin(yawd)*yawd_2dot, -sin(yawd)*yawd_dot^2+cos(yawd)*yawd_2dot, 0]';
% 
% ybd_2dot_1 = ((hat_optr(zbd_2dot)*xcd + hat_optr(zbd)*xcd_2dot)*norm(hat_optr(zbd)*xcd)-...
%              zbd_x_xcd_dot*zbd_xcd_norm_dot)/norm(hat_optr(zbd)*xcd)^2;
% 
% zbd_x_xcd_2dot = hat_optr(zbd_2dot)*xcd + 2*hat_optr(zbd_dot)*xcd_dot + hat_optr(zbd)*xcd_2dot;
% zbd_xcd_norm_2dot = ((zbd_x_xcd_dot'*zbd_x_xcd_dot + (hat_optr(zbd)*xcd)'*zbd_x_xcd_2dot)*norm(hat_optr(zbd)*xcd)-...
%                     ((hat_optr(zbd)*xcd)'*zbd_x_xcd_dot)*zbd_xcd_norm_dot)/norm(hat_optr(zbd)*xcd)^2;
%                 
% ybd_2dot_2 = ((zbd_x_xcd_dot*zbd_xcd_norm_dot + hat_optr(zbd)*xcd*zbd_xcd_norm_2dot)*norm(hat_optr(zbd)*xcd)^2-...
%               2*hat_optr(zbd)*xcd*norm(hat_optr(zbd)*xcd)*zbd_xcd_norm_dot^2)/norm(hat_optr(zbd)*xcd)^4;
%           
% ybd_2dot = ybd_2dot_1 - ybd_2dot_2;
% 
% xbd_2dot = hat_optr(ybd_2dot)*zbd + 2*hat_optr(ybd_dot)*zbd_dot + hat_optr(ybd)*zbd_2dot;
% 
% Rd_2dot = [xbd_2dot ybd_2dot zbd_2dot];
% wd_dot_hat = Rd_dot'*Rd_dot + Rd'*Rd_2dot;
% wd_dot = vee_optr(wd_dot_hat);
% 
% % Moment
% %M = -KR*eR -K_omega*ew + hat_optr(current_omega)*J*current_omega -J*(hat_optr(current_omega)*R'*Rd*wd - R'*Rd*wd_dot);
% M = -KR*eR -K_omega*ew;
% u2 = M(1);u3 = M(2); u4 = M(3);

== matlab function test_without_actuator/MATLAB Function6 ==
  data: qw input; R1 output; qx input; qy input; qz input; R2 output; R3 output
function [R1, R2, R3] = quaternion_to_euler(qw, qx, qy, qz)
    R = qToR(qw,qx,qy,qz);
    R1 = R(:,1);
    R2 = R(:,2);
    R3 = R(:,3);
end

== matlab function test_without_actuator/MATLAB Function7 ==
  data: position input; current_state output size=13; velocity input; qw input; qx input; qy input; qz input; angular_velocity input
function current_state = generate_current_state(position, velocity, qw, qx, qy, qz, angular_velocity)
    % position: 1x3 向量 [x, y, z]
    % velocity: 1x3 向量 [vx, vy, vz]
    % roll: 标量
    % pitch: 标量
    % yaw: 标量
    % angular_velocity: 1x3 向量 [ωx, ωy, ωz]
    
    % 确保所有输入都是列向量
    position = position(:); % 将 position 转换为列向量
    velocity = velocity(:); % 将 velocity 转换为列向量
    angular_velocity = angular_velocity(:); % 将 angular_velocity 转换为列向量
    
    qw = qw(:); % 将 qw 转换为列向量
    qx = qx(:); % 将 qx 转换为列向量
    qy = qy(:); % 将 qy 转换为列向量
    qz = qz(:); % 将 qz 转换为列向量

    % 生成列向量 current_state
    current_state = [position; velocity; qw; qx; qy; qz; angular_velocity];
end

== matlab function test_without_actuator/MATLAB Function8 ==
  data: pos input; desired_state output Bus: desired_state_bus; vel input; acc input; jerk input; snap input; yaw input; yawdot input; yawddot input
function desired_state = generate_desired_state(pos, vel, acc, jerk, snap, yaw, yawdot, yawddot)
    % pos: 1x3 向量 [x_d, y_d, z_d]
    % vel: 1x3 向量 [vx_d, vy_d, vz_d]
    % acc: 1x3 向量 [ax_d, ay_d, az_d]
    % jerk: 1x3 向量 [jerk_x, jerk_y, jerk_z]
    % snap: 1x3 向量 [snap_x, snap_y, snap_z]
    % yaw: 标量
    % yawdot: 标量
    % yawddot: 标量
    
    % 生成结构体 desired_state
    desired_state.pos = pos;
    desired_state.vel = vel;
    desired_state.acc = acc;
    desired_state.jerk = jerk;
    desired_state.snap = snap;
    desired_state.yaw = yaw;
    desired_state.yawdot = yawdot;
    desired_state.yawddot = yawddot;
    %disp('fuck1')
end

== matlab function test_without_actuator/MATLAB Function9 ==
  data: x input; position output; y input; z input
function position = calculate_position(x, y, z)
    % 创建包含 x、y 和 z 坐标的位置向量
    position = [x, y, z];
end

== matlab function test_without_actuator/MATLAB Function10 ==
  data: Kp input; K output Bus: K_bus; Kv input; KR input; K_omega input
function K = generate_K(Kp, Kv, KR, K_omega)
    % 生成一个包含控制增益对角矩阵的结构体
    % Kp: 位置控制的比例增益，3维向量
    % Kv: 速度控制的比例增益，3维向量
    % KR: 角度控制的比例增益，3维向量
    % K_omega: 角速度控制的比例增益，3维向量
    % 定义输出结构体K的字段大小
    K.Kp = zeros(3, 3);
    K.Kv = zeros(3, 3);
    K.KR = zeros(3, 3);
    K.K_omega = zeros(3, 3);
    
    % 创建对角矩阵并赋值给结构体
    K.Kp = diag(Kp(:));
    K.Kv = diag(Kv(:));
    K.KR = diag(KR(:));
    K.K_omega = diag(K_omega(:));
end

== matlab function test_without_actuator/MATLAB Function11 ==
  data: qw input; yaw output; qx input; qy input; qz input
function yaw = quaternionToYaw(qw, qx, qy, qz)
    % 计算yaw角
    % 输入参数为四元数的四个分量：qw, qx, qy, qz
    % 输出为yaw角，单位为弧度
    
    % 使用四元数到欧拉角的转换公式计算yaw角
    siny_cosp = 2 * (qw * qz + qx * qy);
    cosy_cosp = 1 - 2 * (qy * qy + qz * qz);
    yaw = atan2(siny_cosp, cosy_cosp);
end

== matlab function test_without_actuator/MATLAB Function12 ==
  data: trajectory input; pos output; vel output; acc output; jerk output; snap output; yaw output; yawdot output; yawddot output; prev_pos input; prev_vel input; prev_acc input; prev_jerk input; updated_prev_pos output; updated_prev_vel output; updated_prev_acc output; updated_prev_jerk output
function [pos, vel, acc, jerk, snap, yaw, yawdot, yawddot, updated_prev_pos, updated_prev_vel, updated_prev_acc, updated_prev_jerk] = process_trajectory(trajectory, prev_pos, prev_vel, prev_acc, prev_jerk)
    % trajectory: 1x4 向量，表示一个时刻的 [x, y, z, yaw] 坐标

    % 当前时刻的位置和 yaw
    pos = trajectory(1:3)';
    yaw = trajectory(4);
    % 时间步长 (假设为 0.1，如果不同请调整)
    dt = 0.1;
    
    % 计算速度、加速度、jerk 和 snap
    vel = (pos - prev_pos) / dt;
    acc = (vel - prev_vel) / dt;
    jerk = (acc - prev_acc) / dt;
    snap = (jerk - prev_jerk) / dt;

    % 更新上一时刻的数据
    updated_prev_pos = pos;
    updated_prev_vel = vel;
    updated_prev_acc = acc;
    updated_prev_jerk = jerk;
    
    % 由于 yaw 始终为 0，yaw 的导数也全为 0
    yawdot = 0;
    yawddot = 0;
end

== matlab function test_without_actuator/MATLAB Function13 ==
  data: x input; trajectory output; y input; z input; yaw input
function trajectory = calculate_position(x, y, z, yaw)
    % 创建包含 x、y 和 z 坐标的位置向量
    trajectory = [x, y, z, yaw];
end

== matlab function test_without_actuator/MATLAB Function14 ==
  data: f input; w1 output; tau_x input; tau_y input; w2 output; w3 output; tau_z input; w4 output; C_T input; C_M input; p input; D_p input; D input; Eta input
function [w1, w2, w3, w4] = converter(f, tau_x, tau_y, tau_z, C_T, C_M, p, D_p, D, Eta)
w1 = 0;
w2 = 0;
w3 = 0;
w4 = 0;
if Eta == 1
    % Convert thrust and torque to motor speeds
    % Required parameters: thrust coefficient C_T, torque coefficient C_M, air density ρ, propeller diameter D_p,
    % UAV arm length D, maximum thrust f_max, maximum torque tau_max
     f;
     tau_x
     tau_y
     tau_z
    
    a = [f; tau_x; tau_y; tau_z];
    
    %A = [C_T*p*D_p^4/(4*pi^2), C_T*p*D_p^4/(4*pi^2), C_T*p*D_p^4/(4*pi^2), C_T*p*D_p^4/(4*pi^2); 
    %   sqrt(2)/2*D*C_T*p*D_p^4/(4*pi^2), -sqrt(2)/2*D*C_T*p*D_p^4/(4*pi^2), -sqrt(2)/2*D*C_T*p*D_p^4/(4*pi^2), sqrt(2)/2*D*C_T*p*D_p^4/(4*pi^2);
    %    sqrt(2)/2*D*C_T*p*D_p^4/(4*pi^2), sqrt(2)/2*D*C_T*p*D_p^4/(4*pi^2), -sqrt(2)/2*D*C_T*p*D_p^4/(4*pi^2), -sqrt(2)/2*D*C_T*p*D_p^4/(4*pi^2);
    %    C_M*p*D_p^5/(4*pi^2), -C_M*p*D_p^5/(4*pi^2), C_M*p*D_p^5/(4*pi^2), -C_M*p*D_p^5/(4*pi^2)];
    KF = C_T*p*D_p^4/(4*pi^2);
    KM = C_M*p*D_p^5/(4*pi^2);
    A = [KF, KF, KF, KF;
        0, KF*D, 0, -KF*D;
        -KF*D, 0, KF*D, 0;
        KM, -KM, KM, -KM];
    
    
    b = A\a;%表达式 A\b 用于求解方程 Ax=b中的未知向量x
    %disp('fuck')
    %b(b < 0) = 0;
    % 期望的f的大小方向不管Eta怎么规划的，都应是不变的，随着Eta改变的是产生f的方式
    % 根据Eta处理转速,跟Eta无关
    % 计算实际的转速
    w1 = sqrt(b(1))
    w2 = sqrt(b(2))
    w3 = sqrt(b(3))
    w4 = sqrt(b(4))
end
%初始姿态绕x轴转了pi
if Eta == -1
    % Convert thrust and torque to motor speeds
    % Required parameters: thrust coefficient C_T, torque coefficient C_M, air density ρ, propeller diameter D_p,
    % UAV arm length D, maximum thrust f_max, maximum torque tau_max
     f = f;
     tau_x;
     tau_y;
     tau_z;
    
    a = [f; tau_x; tau_y; tau_z];
    
    %A = [C_T*p*D_p^4/(4*pi^2), C_T*p*D_p^4/(4*pi^2), C_T*p*D_p^4/(4*pi^2), C_T*p*D_p^4/(4*pi^2); 
    %   sqrt(2)/2*D*C_T*p*D_p^4/(4*pi^2), -sqrt(2)/2*D*C_T*p*D_p^4/(4*pi^2), -sqrt(2)/2*D*C_T*p*D_p^4/(4*pi^2), sqrt(2)/2*D*C_T*p*D_p^4/(4*pi^2);
    %    sqrt(2)/2*D*C_T*p*D_p^4/(4*pi^2), sqrt(2)/2*D*C_T*p*D_p^4/(4*pi^2), -sqrt(2)/2*D*C_T*p*D_p^4/(4*pi^2), -sqrt(2)/2*D*C_T*p*D_p^4/(4*pi^2);
    %    C_M*p*D_p^5/(4*pi^2), -C_M*p*D_p^5/(4*pi^2), C_M*p*D_p^5/(4*pi^2), -C_M*p*D_p^5/(4*pi^2)];
    KF = C_T*p*D_p^4/(4*pi^2);
    KM = C_M*p*D_p^5/(4*pi^2);
    A = [KF, KF, KF, KF;
        0, -KF*D, 0, KF*D;
        -KF*D, 0, KF*D, 0;
        KM, -KM, KM, -KM];
    
    
    b = A\a;%表达式 A\b 用于求解方程 Ax=b中的未知向量x
    %disp('fuck')
    %b(b < 0) = 0;
    % 期望的f的大小方向不管Eta怎么规划的，都应是不变的，随着Eta改变的是产生f的方式
    % 根据Eta处理转速,跟Eta无关
    % 计算实际的转速
    w1 = -sqrt(b(1));
    w2 = -sqrt(b(2));
    w3 = -sqrt(b(3));
    w4 = -sqrt(b(4));
end

end

== matlab function test_without_actuator/混合无人机模型2/Quadcopter Dynamics Model/Control Effectiveness Model/MATLAB Function ==
  data: w1 input; f output; w2 input; w3 input; w4 input; c_T input; c_M input; d input; tau_x output; tau_y output; tau_z output; p input; Eta input
function [f, tau_x, tau_y, tau_z] = fcn(w1, w2, w3, w4, c_T, c_M, d, p, Eta)
% 函数描述
% 1.作用：本函数用来计算螺旋桨旋转产生的总拉力和反扭力矩。
% 2.函数输入：
%   wi：四个螺旋桨的转速(rad/s)，可以为正或负
%   c_T：螺旋桨拉力系数和外面的converter的CT不同，已经经过换算就等于KF
%   c_M：螺旋桨转矩系数= KM
%   d：机体中心和任一电机的距离(m)
% 3.函数输出：
%   f：螺旋桨拉力（机体轴）
%   tau_x：x轴反扭力矩（机体轴）
%   tau_y：y轴反扭力矩（机体轴）
%   tau_z：z轴反扭力矩（机体轴）
% 4.四旋翼构型为"+”型，螺旋桨序号如下所示：
%            y
%            2↑
%            |
%        3↓—— —— 1↓   x
%            |
%            4↑
f=w1;tau_x=w2;tau_y=w3;tau_z=w4;
if Eta == 1
    f=w1;tau_x=w2;tau_y=w3;tau_z=w4;
end

if Eta == -1
    f=-w1;tau_x=w2;tau_y=w3;tau_z=w4;
end

== matlab function test_without_actuator/混合无人机模型1/Quadcopter Dynamics Model/Control Effectiveness Model/MATLAB Function ==
  data: w1 input; f output; w2 input; w3 input; w4 input; c_T input; c_M input; d input; tau_x output; tau_y output; tau_z output; p input; Eta input
function [f, tau_x, tau_y, tau_z] = fcn(w1, w2, w3, w4, c_T, c_M, d, p, Eta)
% 函数描述
% 1.作用：本函数用来计算螺旋桨旋转产生的总拉力和反扭力矩。
% 2.函数输入：
%   wi：四个螺旋桨的转速(rad/s)，可以为正或负
%   c_T：螺旋桨拉力系数和外面的converter的CT不同，已经经过换算就等于KF
%   c_M：螺旋桨转矩系数= KM
%   d：机体中心和任一电机的距离(m)
% 3.函数输出：
%   f：螺旋桨拉力（机体轴）
%   tau_x：x轴反扭力矩（机体轴）
%   tau_y：y轴反扭力矩（机体轴）
%   tau_z：z轴反扭力矩（机体轴）
% 4.四旋翼构型为"+”型，螺旋桨序号如下所示：
%            y
%            2↑
%            |
%        3↓—— —— 1↓   x
%            |
%            4↑
f=w1;tau_x=w2;tau_y=w3;tau_z=w4;
if Eta == 1
    f=w1;tau_x=w2;tau_y=w3;tau_z=w4;
end

if Eta == -1
    %f=-w1;tau_x=w2;tau_y=w3;tau_z=w4;
    f=w1;tau_x=w2;tau_y=w3;tau_z=w4;
end

== matlab function test_without_actuator/混合无人机模型1/Quadcopter Dynamics Model/MATLAB Function ==
  data: x input; density output; y input
function density = air_density(x, y)
    % 定义火坑的中心位置
    center_x = 10;
    center_y = 10;

    % 定义火坑的半径
    radius = 0.00001;

    % 定义火坑中心的空气密度为1.078 kg/m³
    density_center = 1.078;

    % 定义火坑边缘的空气密度为日常密度值
    density_edge = 1.225;

    % 计算无人机到火坑中心的距离
    r = sqrt((x - center_x)^2 + (y - center_y)^2);

    % 定义高斯函数的标准差
    sigma = radius / 3;
    
    % 使用高斯函数计算空气密度
    density = density_edge + (density_center - density_edge) * exp(-(r.^2) / (2 * sigma^2));


    density = density/1.225;
end

== matlab function test_without_actuator/混合无人机模型1/Quadcopter Dynamics Model/Rigid-Body Dynamic Model/Attitude Dynamic Model/MATLAB Function ==
  data: tau_x input; p_dot output; tau_y input; tau_z input; w1 input; w2 input; w3 input; w4 input; I_xx input; I_yy input; I_zz input; J_RP input; p input; q input; r input; q_dot output; r_dot output
function [p_dot, q_dot, r_dot] = fcn(tau_x, tau_y, tau_z, w1, w2, w3, w4, I_xx, I_yy, I_zz, J_RP, p, q, r)
% 函数描述
% 1.作用：本函数为四旋翼的姿态动力学微分方程组，通过四旋翼所受力矩和螺旋
%         桨转速计算得到四旋翼的机体角速度
% 2.函数输入：
%   wi：四个螺旋桨的转速(rad/s)
%   tau_x：x轴反扭力矩（机体轴）(N·m)
%   tau_y：y轴反扭力矩（机体轴）(N·m)
%   tau_z：z轴反扭力矩（机体轴）(N·m)
%   I_xx：四旋翼x轴转动惯量(kg·m^2)
%   I_yy：四旋翼y轴转动惯量(kg·m^2)
%   I_zz：四旋翼z轴转动惯量(kg·m^2)
%   J_RP：整个电机转子和螺旋桨绕转轴的总转动惯量(kg·m^2)
%   p：四旋翼x轴角速度（机体轴)(rad/s)
%   q：四旋翼y轴角速度（机体轴)(rad/s)
%   r：四旋翼z轴角速度（机体轴)(rad/s)
% 3.函数输出：
%   p_dot：四旋翼x轴角加速度（机体轴)
%   q_dot：四旋翼y轴角加速度（机体轴)
%   r_dot：四旋翼z轴角加速度（机体轴)
% 4.四旋翼构型为“X”型，螺旋桨序号如下所示：
%            y
%            2↑
%            |
%        3↓—— —— 1↓   x
%            |
%            4↑
%   其中，↑表示螺旋桨逆时针旋转；↓表示螺旋桨顺时针旋转。


p_dot = (1/I_xx) * (tau_x + q * r * (I_yy - I_zz) );
q_dot = (1/I_yy) * (tau_y + p * r * (I_zz - I_xx) );
r_dot = (1/I_zz) * (tau_z + p * q * (I_xx - I_yy) );
end
